simulink model "mfcStairs"  (R2015a)
settings: Solver=ode15s  StartTime=0.0  StopTime=Tsim  RelTol=1e-9  AbsTol=1e-12
InitFcn:
  | delta = 20;
  | kmu = 20000;
  | 
  | beta = 0;
  | %beta = -10;
  | gamma = 0;
  | gamma = 5;
  | 
  | dummy = 0;
  | 
  | mfcInit = [7.01283002283551 487.411110543117 0.98999246131829 0.0499770097528264];
  | 
  | Rinit = 100;
  | Tsim = 6000;
  | res = 1000;
  | tStairs = 0:res:Tsim;
  | ampStairs = zeros(length(tStairs), 1);
  | for i = 1:length(tStairs)
  | ampStairs(i) = Rinit + (i - 1)*5;
  | end
libraries: simulink x1
settings Model: Creator=ironi  LastModifiedBy=ironi
settings HardwareCC: ProdBitPerLong=64  ProdBitPerPointer=64  ProdWordSize=64  ProdHWDeviceType=Generic->64-bit Embedded Processor (LP64)

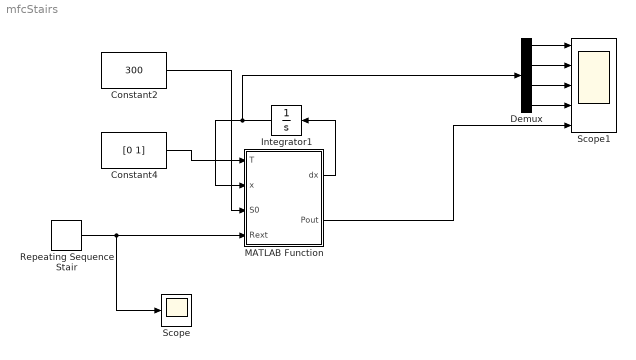
== system mfcStairs ==
  Constant2 : Constant  Value=300
  Constant4 : Constant  Value=[0 1]
  Demux : Demux
  Integrator1 : Integrator  InitialCondition=mfcInit
  MATLAB Function : MATLAB Function  TreatAsAtomicUnit=on
  Repeating Sequence Stair : simulink/Sources/Repeating Sequence Stair  OutValues=ampStairs  tsamp=res  OutMin=[]  OutMax=[]  OutDataTypeStr=double  OutputDataTypeScalingMode=double  OutDataType=fixdt(0,8)  ConRadixGroup=Best Precision: Vector-wise  OutScaling=2^-12
  Scope : Scope
  Scope1 : Scope  NumInputPorts=5
      settings: YMin=-5~-5~-5~-5~-5  YMax=5~5~5~5~5  SaveName=data
  wires:
  MATLAB Function/1(dx) -> Integrator1/1
  Integrator1/1 -> Demux/1, MATLAB Function/2(x)
  Constant4/1 -> MATLAB Function/1(T)
  Constant2/1 -> MATLAB Function/3(S0)
  Demux/2 -> Scope1/2
  Demux/1 -> Scope1/1
  Demux/3 -> Scope1/3
  Demux/4 -> Scope1/4
  MATLAB Function/2(Pout) -> Scope1/5
  Repeating Sequence Stair/1 -> MATLAB Function/4(Rext), Scope/1

== matlab function mfcStairs/MATLAB Function ==
  data: T input; dx output; x input; dummy parameter; S0 input; Rext input; Pout output
function [dx, Pout]= mfcModel(T, x, dummy, S0, Rext)
F = 96485;
R = 8.314472;
T = 298.15;
Y = 22.753;
Ych4 = .3;
qmax_a = 8.48;
qmax_m = 8.2;
umax_a = 1.9753;
umax_m = .1;
Ks_a = 20;
Ks_m = 80;
m = 2;
gamma = 663400;
Mtotal = .05;
Km = .2*Mtotal;
Kd_a = .02*umax_a;
Kd_m = .02*umax_m;
Xmax_a = 512.5;
Xmax_m = 537.5;
Kx = .04;
Rmin = 25;
Rmax = 2000 + Rmin;
Emin = .01;
Emax = 0.25 + 0.4144+ Emin;
Kr = .024;

i0ref=0.4*4;

e = 0.0001*Mtotal;

V = 0.05;
Fin = 0.1527;

D = Fin/V;

S   = x(1);
xa  = x(2);
xm  = x(3);
Mox = x(4);

%% Équations dynamiques
  
Mred = Mtotal - Mox;
% if Mred < 0
%   Mred
% end

Rint = Rmin + (Rmax - Rmin) * exp(-Kr*xa);                          % (22)
Eocv = Emin + (Emax - Emin) * exp(-1/(Kr*xa));                      % (23)

alpha_a = 1/2*(1 + tanh(Kx*(xa + xm - Xmax_a)));                    % (9)
alpha_m = 1/2*(1 + tanh(Kx*(xa + xm - Xmax_m)));                    % (9)

qa = qmax_a * S / (Ks_a + S) * Mox / (Km + Mox);                    % (15)
qm = qmax_m * S / (Ks_m + S);                                       % (16)

ua = umax_a * S / (Ks_a + S) * Mox / (Km + Mox);                    % (13)
um = umax_m * S / (Ks_m + S);                                       % (14)

n_conc = R*T/F/m * log(Mtotal/Mred);                                % (18)

Imfc = (Eocv - n_conc) / (Rext + Rint) * Mred / (e + Mred);         % (21)

Sp = -qa*xa - qm*xm + D*(S0 - S);                                   % (6)
Xap = ua*xa - Kd_a*xa - alpha_a*D*xa;                               % (7)
Xmp = um*xm - Kd_m*xm - alpha_m*D*xm;                               % (8)

Moxp = -Y*qa + gamma*Imfc / (m*F*V*xa) * 86400;                     % (12)

if xa < 1 && Xap < 0
  Xap = 0;
end

if xm < 0.99 && Xmp < 0
  Xmp = 0;
end

% if Mox > Mtotal - 0.0001 && Moxp > 0
%   Moxp = 0;
% end

Pout = Rext*Imfc^2;

dx = [Sp; Xap; Xmp; Moxp];
